simulink model "riggs_model"  (R2023a)
settings: Solver=VariableStepAuto  StartTime=0.0  StopTime=300  RelTol=1e-3
libraries: simulink x1
settings Model: Creator=SAT  LastModifiedBy=User
settings OptimizationCC: ReuseModelBlockBuffer=off
settings DebuggingCC: UnconnectedInputMsg=warning  UnconnectedOutputMsg=warning  UnconnectedLineMsg=warning
settings ModelReferenceCC: EnableRefExpFcnMdlSchedulingChecks=on
settings RTWCC: DLArmComputeVersion=19.05

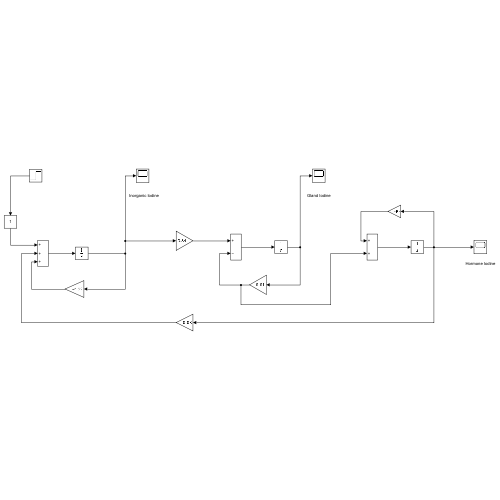
[thumbnail: Simulink's stored preview of the top-level diagram]
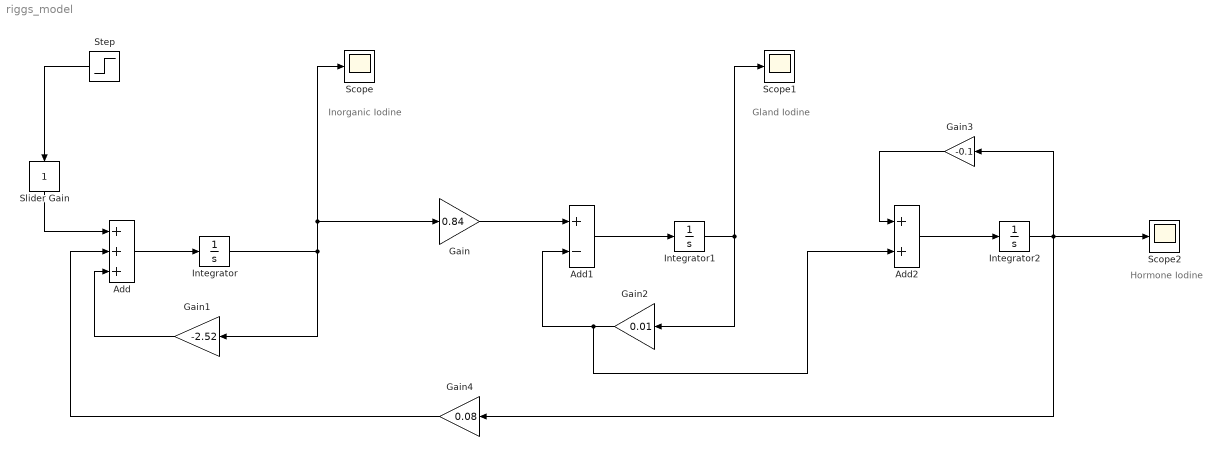
== system riggs_model ==
  note: Inorganic Iodine
  note: Gland Iodine
  note: Hormone Iodine
  Add : Sum  Inputs=+++
  Add1 : Sum  Inputs=+-
  Add2 : Sum
  Gain : Gain  Gain=0.84
  Gain1 : Gain  Gain=-2.52
  Gain2 : Gain  Gain=0.01
  Gain3 : Gain  Gain=-0.1
  Gain4 : Gain  Gain=0.08
  Integrator : Integrator  InitialCondition=81.2
  Integrator1 : Integrator  InitialCondition=6821
  Integrator2 : Integrator  InitialCondition=682
  Scope : Scope
  Scope1 : Scope
  Scope2 : Scope
  Slider Gain : simulink/Math Operations/Slider Gain  gain=1  low=0  high=16
  Step : Step  Before=15  After=15  SampleTime=0
  wires:
  Step/1 -> Slider Gain/1
  Slider Gain/1 -> Add/1
  Add/1 -> Integrator/1
  Integrator/1 -> Scope/1, Gain/1, Gain1/1
  Gain/1 -> Add1/1
  Gain1/1 -> Add/3
  Add1/1 -> Integrator1/1
  Integrator1/1 -> Gain2/1, Scope1/1
  Add2/1 -> Integrator2/1
  Integrator2/1 -> Gain4/1, Scope2/1, Gain3/1
  Gain3/1 -> Add2/1
  Gain4/1 -> Add/2
  Gain2/1 -> Add2/2, Add1/2
